simulink model "demo1"  (R2013b)
settings: Solver=ode45  StartTime=0.0  StopTime=10  RelTol=1e-3
settings Model: Creator=Administrator  LastModifiedBy=Administrator

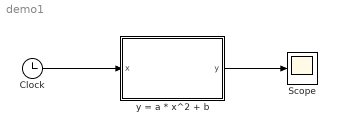
== system demo1 ==
  Clock : Clock
  Scope : Scope
      settings: YMin=-2.56128e+10  YMax=-2.56095e+10
  y = a * x^2 + b : Subsystem  mask(Custom){g_a=1, g_b=20}
      mask prompts: g_a "a"; g_b "b"
      mask help: This block supplies a demo of masking.
      mask Help: helpview('xxx.html');
      mask Callback g_a: check_num('g_a');
      mask Callback g_b: check_num('g_b');
      mask Display:
      | %image(imread('01.jpg'),'bottom-right');
      | a = str2num(get_param(gcbh, 'g_a'));
      | b = str2num(get_param(gcbh, 'g_b'));
      | t = 0:0.1:10;
      | plot(t, a * t.^2 + b);
  wires:
  Clock/1 -> y = a * x^2 + b/1(x)
  y = a * x^2 + b/1(y) -> Scope/1

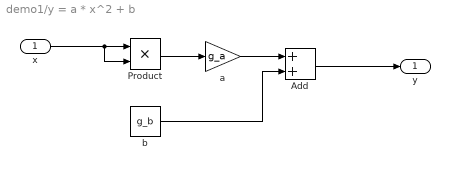
== system demo1/y = a * x^2 + b ==
  x : Inport
  Add : Sum
  Product : Product
  a : Gain  Gain=g_a
  b : Constant  Value=g_b
  y : Outport
  wires:
  x/1 -> Product/2, Product/1
  Product/1 -> a/1
  a/1 -> Add/1
  Add/1 -> y/1
  b/1 -> Add/2
